simulink library "squaredExponentialCovMat_ul"  (R2018b)
settings: Solver=VariableStepAuto  StartTime=0.0  StopTime=10.0  RelTol=1e-3
settings Model: Creator=Ayaz  LastModifiedBy=asiddiq2

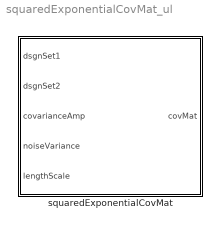
== system squaredExponentialCovMat_ul ==
  squaredExponentialCovMat : Subsystem

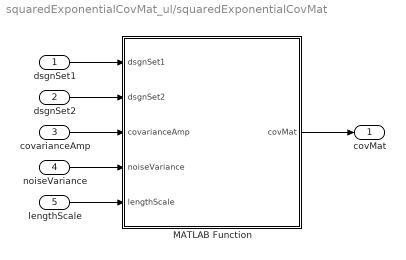
== system squaredExponentialCovMat_ul/squaredExponentialCovMat ==
  dsgnSet1 : Inport
  dsgnSet2 : Inport  Port=2
  covarianceAmp : Inport  Port=3
  noiseVariance : Inport  Port=4
  lengthScale : Inport  Port=5
  MATLAB Function : MATLAB Function  TreatAsAtomicUnit=on
  covMat : Outport
  wires:
  dsgnSet1/1 -> MATLAB Function/1(dsgnSet1)
  lengthScale/1 -> MATLAB Function/5(lengthScale)
  MATLAB Function/1(covMat) -> covMat/1
  dsgnSet2/1 -> MATLAB Function/2(dsgnSet2)
  covarianceAmp/1 -> MATLAB Function/3(covarianceAmp)
  noiseVariance/1 -> MATLAB Function/4(noiseVariance)

== matlab function squaredExponentialCovMat_ul/squaredExponentialCovMat/MATLAB Function ==
  data: dsgnSet1 input; covMat output; dsgnSet2 input; covarianceAmp input; noiseVariance input; lengthScale input
function covMat = buildCovarianceMatrix(dsgnSet1,dsgnSet2,covarianceAmp,noiseVariance,lengthScale)

% function that builds covariance matrix between design sets
% inputs datapoints, covariance amplitude, noise variance and length scale

% length scale quantifies the relevance of the components in the input
% vector for predicting the outputs

% covariance formula
cov = @(x1,x2,covAmp,noiseVar,lengthScl)...
    covAmp*(exp(-0.5*((x1-x2)'*(eye(numel(lengthScl))./(lengthScl.^2))*(x1-x2))));

% convariance matrix size
covMatSize = [size(dsgnSet1,2), size(dsgnSet2,2)];
covMat = zeros(covMatSize);

if isequal(dsgnSet1,dsgnSet2)
    for ii = 1:covMatSize(1)
        for jj = ii:covMatSize(2)
            covMat(ii,jj) = cov(dsgnSet1(:,ii),dsgnSet2(:,jj),...
                covarianceAmp,noiseVariance,lengthScale);
            
        end
    end
    covMat = covMat + covMat' - eye(length(covMat)).*diag(covMat - noiseVariance);
    
else
    for ii = 1:covMatSize(1)
        for jj = 1:covMatSize(2)
            covMat(ii,jj) = cov(dsgnSet1(:,ii),dsgnSet2(:,jj),...
                covarianceAmp,noiseVariance,lengthScale);
        end
    end
end

end
